simulink model "W05_SteadyStateError"  (R2024b)
settings: Solver=ode45  StartTime=0.0  StopTime=t_end  MaxStep=0.005  RelTol=1e-3
PreLoadFcn:
  | % W05_SteadyStateError 기본 파라미터 (모델을 열 때 자동 실행)
  | % 기본값은 Ki = 0 : 비례제어만 -> 정상상태 오차가 남는 것을 보여 줍니다.
  | defs = { 'Kp',50 ; 'Ki',0 ; 'r_amp',10 ; 't_end',5 ;
  |          'numG',0.01 ; 'denG',[0.005 0.06 0.1001] };
  | for ii = 1:size(defs,1)
  |     if ~evalin('base', sprintf('exist(''%s'',''var'')', defs{ii,1}))
  |         assignin('base', defs{ii,1}, defs{ii,2});
  |     end
  | end
  | clear defs ii
values from neighbouring files (symbols this model uses):
  Ki = Ki_max*1.2    [W05_03_run_simulink.m]
  Kp = dcgain(Ls{i})    [W05_02_steady_state_error.m]    (also in W05_03_run_simulink.m = 50)
  r_amp = 10    [W05_03_run_simulink.m]
undefined symbols (not defined in the file or in its folder): denG, numG
settings Model: Creator=admin  LastModifiedBy=admin

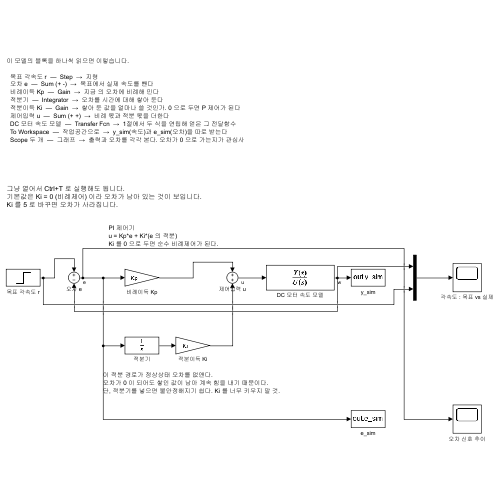
[thumbnail: Simulink's stored preview of the top-level diagram]
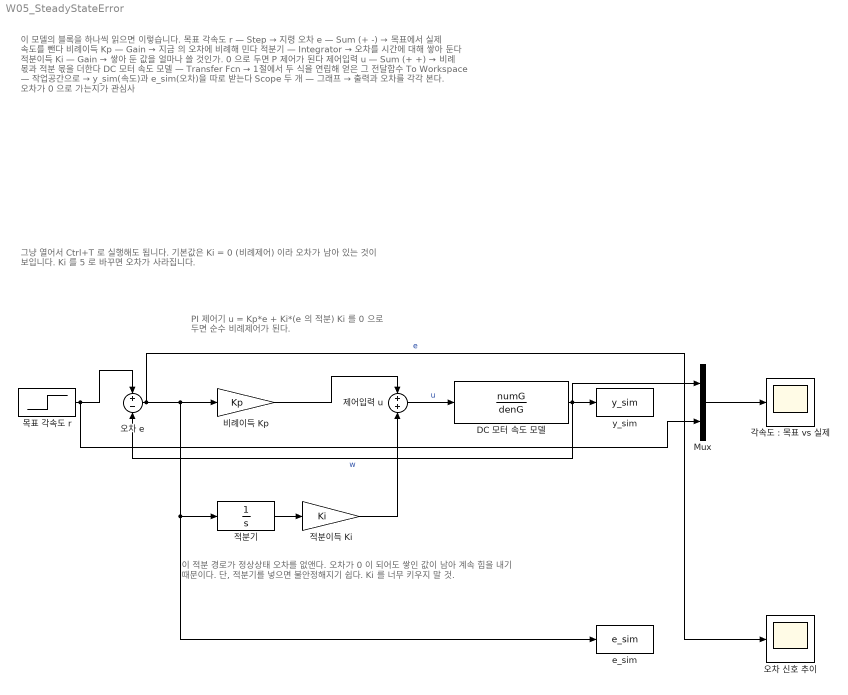
== system W05_SteadyStateError ==
  note: PI 제어기
      | u = Kp*e + Ki*(e 의 적분)
      | Ki 를 0 으로 두면 순수 비례제어가 된다.
  note: 이 적분 경로가 정상상태 오차를 없앤다.
      | 오차가 0 이 되어도 쌓인 값이 남아 계속 힘을 내기 때문이다.
      | 단, 적분기를 넣으면 불안정해지기 쉽다. Ki 를 너무 키우지 말 것.
  note: 그냥 열어서 Ctrl+T 로 실행해도 됩니다.
      | 기본값은 Ki = 0 (비례제어) 이라 오차가 남아 있는 것이 보입니다.
      | Ki 를 5 로 바꾸면 오차가 사라집니다.
  note: 이 모델의 블록을 하나씩 읽으면 이렇습니다.
      |
      |   목표 각속도 r  —  Step  →  지령
      |   오차 e  —  Sum (+ -)  →  목표에서 실제 속도를 뺀다
      |   비례이득 Kp  —  Gain  →  지금 의 오차에 비례해 민다
      |   적분기  —  Integrator  →  오차를 시간에 대해 쌓아 둔다
      |   적분이득 Ki  —  Gain  →  쌓아 둔 값을 얼마나 쓸 것인가. 0 으로 두면 P 제어가 된다
      |   제어입력 u  —  Sum (+ +)  →  비례 몫과 적분 몫을 더한다
      |   DC 모터 속도 모델  —  Transfer Fcn  →  1절에서 두 식을 연립해 얻은 그 전달함수
      |   To Workspace  —  작업공간으로  →  y_sim(속도)과 e_sim(오차)을 따로 받는다
      |   Scope 두 개  —  그래프  →  출력과 오차를 각각 본다. 오차가 0 으로 가는지가 관심사
  DC 모터 속도 모델 : TransferFcn  Numerator=numG  Denominator=denG
  Mux : Mux  Inputs=2
  e_sim : ToWorkspace  VariableName=e_sim  SaveFormat=Timeseries  SampleTime=-1
  y_sim : ToWorkspace  VariableName=y_sim  SaveFormat=Timeseries  SampleTime=-1
  "각속도 : 목표 vs 실제" : Scope
  목표 각속도 r : Step  Time=0  After=r_amp  SampleTime=0
  비례이득 Kp : Gain  Gain=Kp
  오차 e : Sum  Inputs=+-
  오차 신호 추이 : Scope
  적분기 : Integrator
  적분이득 Ki : Gain  Gain=Ki
  제어입력 u : Sum
  wires:
  목표 각속도 r/1 -> 오차 e/1, Mux/2
  오차 e/1 -> e_sim/1, 적분기/1, 비례이득 Kp/1, 오차 신호 추이/1  "e"
  적분기/1 -> 적분이득 Ki/1
  비례이득 Kp/1 -> 제어입력 u/1
  적분이득 Ki/1 -> 제어입력 u/2
  제어입력 u/1 -> DC 모터 속도 모델/1  "u"
  DC 모터 속도 모델/1 -> y_sim/1, 오차 e/2, Mux/1  "w"
  Mux/1 -> "각속도 : 목표 vs 실제"/1
